simulink model "trans_fun"  (Simulink 7.9)
settings: Solver=ode45  StartTime=0.0  StopTime=10.0  RelTol=1e-3
settings Model: Creator=Nice  LastModifiedBy=Nice

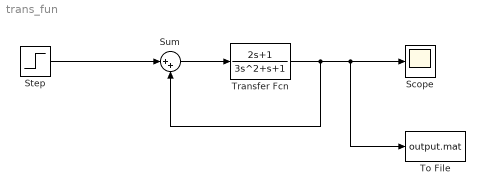
== system trans_fun ==
  Scope : Scope
  Step : Step  SampleTime=0
  Sum : Sum  Inputs=|++
  To File : ToFile  Filename=output.mat  MatrixName=out  SaveFormat=Timeseries
  Transfer Fcn : TransferFcn  Numerator=[2 1]  Denominator=[3 1 1]
  wires:
  Step/1 -> Sum/1
  Sum/1 -> Transfer Fcn/1
  Transfer Fcn/1 -> Sum/2, Scope/1, To File/1
